simulink model "Two_mass_Osillation"  (R2021a)
settings: Solver=FixedStepAuto  StartTime=0.0  StopTime=10  FixedStep=Ts_10k  RelTol=1e-3
values from neighbouring files (symbols this model uses):
  B1 = 0.5*J1    (= 19000)    [Two_mass_oscillation_sim_param_20221213.m]    (also in theoritcal_sim.m)
  B2 = 0.01*J2    (= 38)    [Two_mass_oscillation_sim_param_20221213.m]    (also in theoritcal_sim.m)
  J1 = 38000    [Two_mass_oscillation_sim_param_20221213.m]    (also in theoritcal_sim.m)
  J2 = 0.1*n*J1    (= 3800)    [Two_mass_oscillation_sim_param_20221213.m]    (also in theoritcal_sim.m)
  K = 10*J1    (= 380000)    [Two_mass_oscillation_sim_param_20221213.m]    (also in theoritcal_sim.m)
  Kd_Speed = 0    [Two_mass_oscillation_sim_param_20221213.m]
  Ki_Speed = B1*BW_Speed    (= 11938052.0836)    [Two_mass_oscillation_sim_param_20221213.m]
  Kp_Speed = (J1+J2)*BW_Speed    (= 26263714.584)    [Two_mass_oscillation_sim_param_20221213.m]
  PP = Pole/2    (= 5)    [Two_mass_oscillation_sim_param_20221213.m]
libraries: simulink x2
settings Model: Creator=user  LastModifiedBy=williampai
settings SolverCC: AlgebraicLoopSolver=TrustRegion
settings DebuggingCC: UnconnectedInputMsg=none  UnconnectedOutputMsg=none  UnconnectedLineMsg=none
settings RTWCC: DLArmComputeVersion=20.02.1

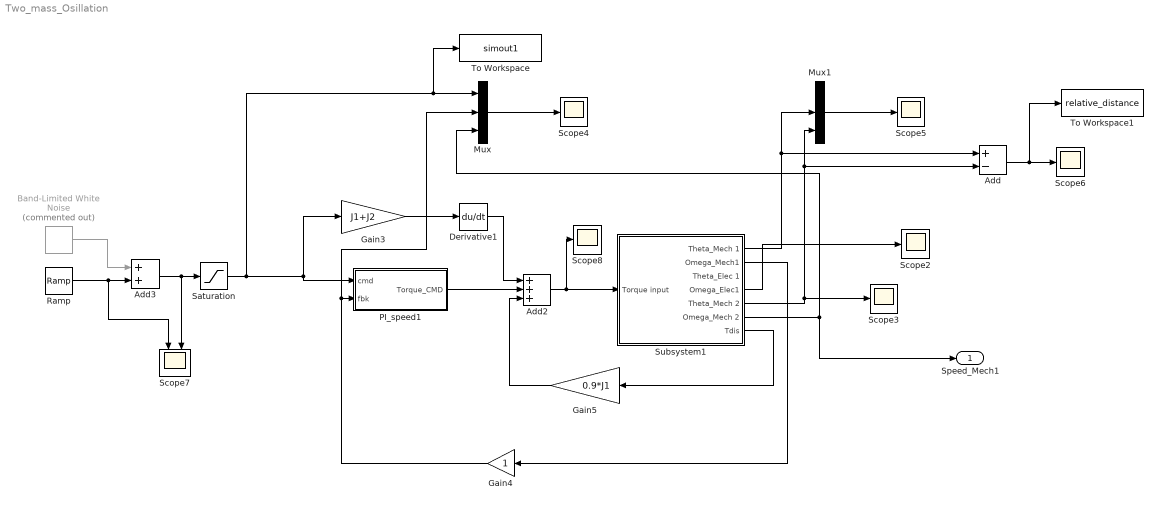
== system Two_mass_Osillation ==
  Add : Sum  Inputs=+-
  Add2 : Sum  Inputs=+++
  Add3 : Sum
  Band-Limited White Noise : simulink/Sources/Band-Limited White Noise  Commented=on  Cov=[0.1]  Ts=0.1  seed=[23341]
  Derivative1 : Derivative
  Gain3 : Gain  Gain=J1+J2
  Gain4 : Gain
  Gain5 : Gain  Gain=0.9*J1
  Mux : Mux  Inputs=3
  Mux1 : Mux  Inputs=3
  PI_speed1 : Subsystem
  Ramp : simulink/Sources/Ramp  slope=9.8  start=0  InitialOutput=0
  Saturation : Saturate  UpperLimit=41.667  LowerLimit=-55
  Scope{2..6,8} (6 alike) : Scope
  Scope7 : Scope  NumInputPorts=2
  Subsystem1 : Subsystem
  To Workspace : ToWorkspace  VariableName=simout1  SaveFormat=Timeseries  SampleTime=-1
  To Workspace1 : ToWorkspace  VariableName=relative_distance  SaveFormat=Timeseries  SampleTime=-1
  Speed_Mech1 : Outport
  wires:
  Add2/1 -> Scope8/1, Subsystem1/1(Torque input)
  Subsystem1/2(Omega_Mech1) -> Gain4/1
  Band-Limited White Noise/1 -> Add3/1
  Add3/1 -> Scope7/2, Saturation/1
  Add/1 -> To Workspace1/1, Scope6/1
  Saturation/1 -> To Workspace/1, Mux/1, Gain3/1, PI_speed1/1(cmd)
  Subsystem1/1(Theta_Mech 1) -> Mux1/2, Add/1
  Mux/1 -> Scope4/1
  Ramp/1 -> Scope7/1, Add3/2
  Subsystem1/5(Theta_Mech 2) -> Mux1/3, Add/2, Scope3/1
  Subsystem1/4(Omega_Elec1) -> Scope2/1
  PI_speed1/1(Torque_CMD) -> Add2/2
  Gain3/1 -> Derivative1/1
  Mux1/1 -> Scope5/1
  Subsystem1/7(Tdis) -> Gain5/1
  Gain4/1 -> Mux/2, PI_speed1/2(fbk)
  Subsystem1/6(Omega_Mech 2) -> Mux/3, Speed_Mech1/1
  Derivative1/1 -> Add2/1
  Gain5/1 -> Add2/3

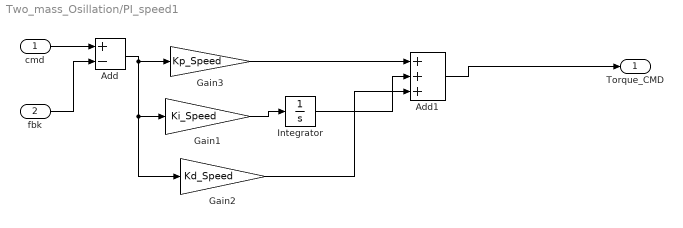
== system Two_mass_Osillation/PI_speed1 ==
  cmd : Inport
  fbk : Inport  Port=2
  Add : Sum  Inputs=+-
  Add1 : Sum  Inputs=+++
  Gain1 : Gain  Gain=Ki_Speed
  Gain2 : Gain  Gain=Kd_Speed
  Gain3 : Gain  Gain=Kp_Speed
  Integrator : Integrator
  Torque_CMD : Outport
  wires:
  Integrator/1 -> Add1/2
  Gain1/1 -> Integrator/1
  Add/1 -> Gain3/1, Gain2/1, Gain1/1
  fbk/1 -> Add/2
  cmd/1 -> Add/1
  Gain3/1 -> Add1/1
  Add1/1 -> Torque_CMD/1
  Gain2/1 -> Add1/3

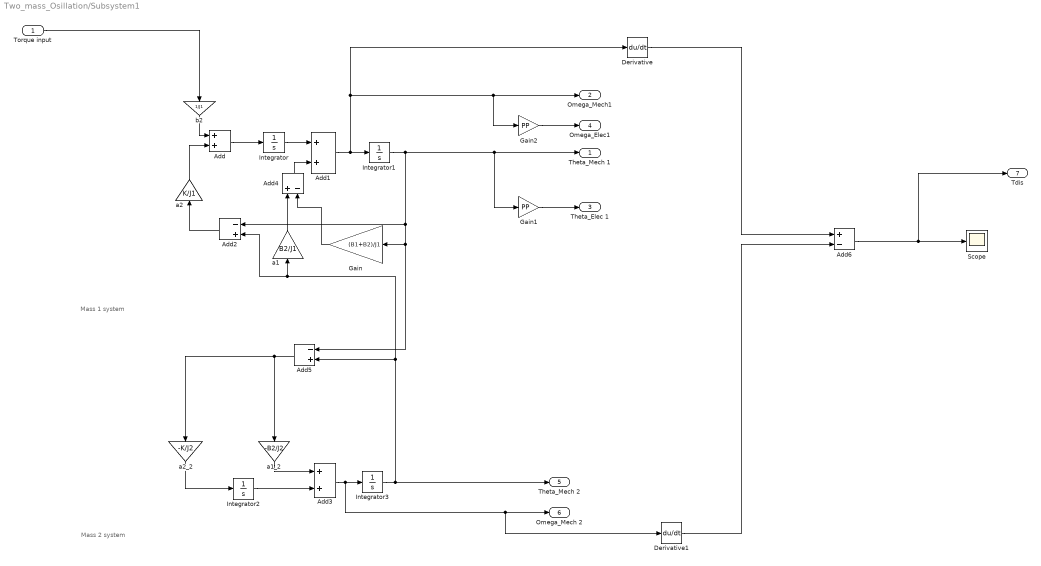
== system Two_mass_Osillation/Subsystem1 ==
  note: Mass 1 system
  note: Mass 2 system
  Torque input : Inport
  Add : Sum
  Add1 : Sum
  Add2 : Sum  Inputs=-+
  Add3 : Sum
  Add4 : Sum  Inputs=+-
  Add5 : Sum  Inputs=-+
  Add6 : Sum  Inputs=+-
  Derivative : Derivative
  Derivative1 : Derivative
  Gain : Gain  Gain=(B1+B2)/J1
  Gain1 : Gain  Gain=PP
  Gain2 : Gain  Gain=PP
  Integrator{,1..3} (4 alike) : Integrator
  Scope : Scope
  a1 : Gain  Gain=B2/J1
  a1_2 : Gain  Gain=-B2/J2
  a2 : Gain  Gain=K/J1
  a2_2 : Gain  Gain=-K/J2
  b2 : Gain  Gain=1/J1
  Theta_Mech 1 : Outport
  Omega_Mech1 : Outport  Port=2
  Theta_Elec 1 : Outport  Port=3
  Omega_Elec1 : Outport  Port=4
  Theta_Mech 2 : Outport  Port=5
  Omega_Mech 2 : Outport  Port=6
  Tdis : Outport  Port=7
  wires:
  Integrator/1 -> Add1/1
  b2/1 -> Add/1
  Integrator1/1 -> Add2/1, Add5/1, Gain/1, Gain1/1, Theta_Mech 1/1
  Integrator2/1 -> Add3/2
  a2/1 -> Add/2
  Add1/1 -> Integrator1/1, Derivative/1, Gain2/1, Omega_Mech1/1
  Add/1 -> Integrator/1
  Add2/1 -> a2/1
  a2_2/1 -> Integrator2/1
  Add4/1 -> Add1/2
  Add5/1 -> a1_2/1, a2_2/1
  a1_2/1 -> Add3/1
  Add3/1 -> Derivative1/1, Omega_Mech 2/1, Integrator3/1
  Integrator3/1 -> Theta_Mech 2/1, Add5/2, Add2/2, a1/1
  Torque input/1 -> b2/1
  Gain1/1 -> Theta_Elec 1/1
  Gain2/1 -> Omega_Elec1/1
  Derivative1/1 -> Add6/2
  Derivative/1 -> Add6/1
  Add6/1 -> Tdis/1, Scope/1
  a1/1 -> Add4/1
  Gain/1 -> Add4/2
